simulink model "kaskada_dir"  (R2015a)
settings: Solver=ode45  StartTime=0.0  StopTime=10.0  RelTol=1e-3
settings Model: Creator=Bojana Vasic  LastModifiedBy=Bojana Vasic

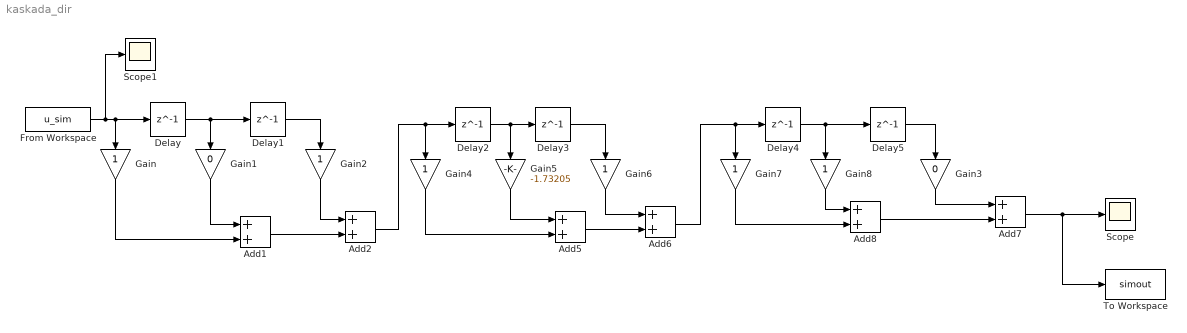
== system kaskada_dir ==
  Add{1..2,5..8} (6 alike) : Sum
  Delay{,1..5} (6 alike) : Delay  DelayLength=1
  From Workspace : FromWorkspace  VariableName=u_sim  SampleTime=1
  Gain{,2,4,6..8} (6 alike) : Gain
  Gain1 : Gain  Gain=0
  Gain3 : Gain  Gain=0
  Gain5 : Gain  Gain=-1.73205
  Scope : Scope
  Scope1 : Scope
  To Workspace : ToWorkspace  VariableName=simout  SaveFormat=Timeseries  SampleTime=-1
  wires:
  From Workspace/1 -> Scope1/1, Delay/1, Gain/1
  Gain/1 -> Add1/2
  Gain1/1 -> Add1/1
  Delay/1 -> Delay1/1, Gain1/1
  Delay1/1 -> Gain2/1
  Gain2/1 -> Add2/1
  Add1/1 -> Add2/2
  Add2/1 -> Gain4/1, Delay2/1
  Delay2/1 -> Gain5/1, Delay3/1
  Gain4/1 -> Add5/2
  Gain5/1 -> Add5/1
  Delay3/1 -> Gain6/1
  Gain6/1 -> Add6/1
  Add5/1 -> Add6/2
  Add6/1 -> Gain7/1, Delay4/1
  Gain7/1 -> Add8/2
  Delay4/1 -> Gain8/1, Delay5/1
  Gain8/1 -> Add8/1
  Delay5/1 -> Gain3/1
  Add8/1 -> Add7/2
  Gain3/1 -> Add7/1
  Add7/1 -> To Workspace/1, Scope/1
